simulink model "UIO_SFControl"  (R2019b)
settings: Solver=VariableStepAuto  StartTime=0.0  StopTime=1500.0  RelTol=1e-3
values from neighbouring files (symbols this model uses):
  A5 = [1 -49.59 -0.4121 4.877 0.1209; 0 0.9835 0.01639 0 0; 0 0 0.9835 0 0 ... (first row only)    [AugmentedRev1.m]    (also in DiscreteSystem.m)
  B5 = [0.85 -0.002296 0.002032; 0 0.0001374 0; 0 0.01653 0; 0 0 0.001209 ... (first row only)    [AugmentedRev1.m]    (also in DiscreteSystem.m)
  C = [1 0 0 0 0]    [AugmentedRev1.m]
  C5 = [1 0 0 0 0; 0 1 0 0 0; 0 0 1 0 0; 0 0 0 1 0; 0 0 0 0 1]    [AugmentedRev1.m]    (also in DiscreteSystem.m)
  C5_c = [1 0 0 0 0; 0 1 0 0 0; 0 0 1 0 0; 0 0 0 1 0; 0 0 0 0 1]    [AugmentedRev1.m]    (also in DiscreteSystem.m)
  D5 = [0 0 0; 0 0 0; 0 0 0; 0 0 0; 0 0 0]    [AugmentedRev1.m]    (also in DiscreteSystem.m)
  F5 = k*[1/th2 -th3 -th3 2 2]    [AugmentedRev1.m]    (also in DiscreteSystem.m)
  L = [0.0048; 0; 0; 0; 0]    [AugmentedRev1.m]
  th1 = 0.85    [AugmentedRev1.m]    (also in DiscreteSystem.m)
  th2 = 50    [AugmentedRev1.m]    (also in DiscreteSystem.m)
  th3 = 60    [AugmentedRev1.m]    (also in DiscreteSystem.m)
undefined symbols (not defined in the file or in its folder): Bu, Bu1
libraries: dspsrcs4 x2
settings Model: Creator=akshita_jain  LastModifiedBy=akshita_jain

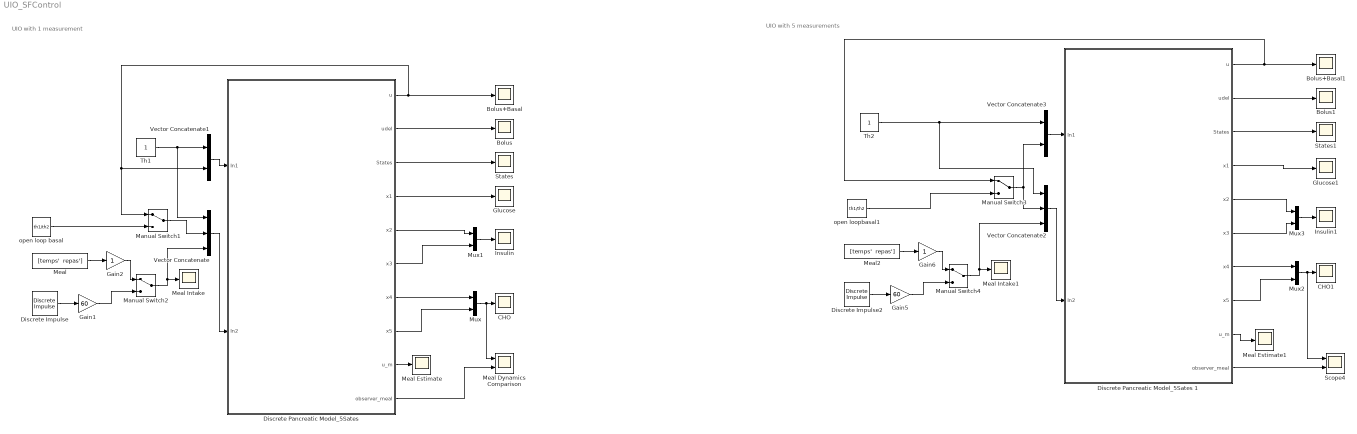
== system UIO_SFControl ==
  note: UIO with 5 measurements
  note: UIO with 1 measurement
  Bolus : Scope
  Bolus+Basal : Scope
  Bolus+Basal1 : Scope
  Bolus1 : Scope
  CHO : Scope
  CHO1 : Scope
  Discrete Impulse : dspsrcs4/Discrete  Impulse  Delay=110  SampleTime=1  FrameSample=1  OutputFrames=off  dataType=double  isSigned=on  wordLen=16  udDataType=sfix(16)  fracBitsMode=Best precision  numFracBits=15  OutDataTypeStr=double  LastOutDataTypeStr=double
  Discrete Impulse2 : dspsrcs4/Discrete  Impulse  Delay=110  SampleTime=1  FrameSample=1  OutputFrames=off  dataType=double  isSigned=on  wordLen=16  udDataType=sfix(16)  fracBitsMode=Best precision  numFracBits=15  OutDataTypeStr=double  LastOutDataTypeStr=double
  "Discrete Pancreatic Model_5Sates " : Subsystem
  Discrete Pancreatic Model_5Sates 1 : Subsystem
  Gain1 : Gain  Gain=60
  Gain2 : Gain
  Gain5 : Gain  Gain=60
  Gain6 : Gain
  Glucose : Scope
  Glucose1 : Scope
  Insulin : Scope
  Insulin1 : Scope
  Manual Switch{1..4} (4 alike) : ManualSwitch
  Meal : FromWorkspace  VariableName="[temps'  repas']"  SampleTime=0
  Meal Dynamics Comparison : Scope  NumInputPorts=2
  Meal Estimate : Scope
  Meal Estimate1 : Scope
  Meal Intake : Scope
  Meal Intake1 : Scope
  Meal2 : FromWorkspace  VariableName="[temps'  repas']"  SampleTime=0
  Mux{,1..3} (4 alike) : Mux  Inputs=2
  Scope4 : Scope  NumInputPorts=2
  States : Scope
  States1 : Scope
  Th1 : Constant
  Th2 : Constant
  Vector Concatenate : Concatenate  NumInputs=3
  Vector Concatenate1 : Concatenate
  Vector Concatenate2 : Concatenate  NumInputs=3
  Vector Concatenate3 : Concatenate
  open loop basal : Constant  Value=th1/th2
  open loopbasal1 : Constant  Value=th1/th2
  wires:
  Manual Switch1/1 -> Vector Concatenate/2
  "Discrete Pancreatic Model_5Sates "/1(u) -> Bolus+Basal/1, Manual Switch1/1, Vector Concatenate1/2
  Th1/1 -> Vector Concatenate/1, Vector Concatenate1/1
  Mux/1 -> Meal Dynamics Comparison/1, CHO/1
  "Discrete Pancreatic Model_5Sates "/4(x1) -> Glucose/1
  Discrete Impulse/1 -> Gain1/1
  "Discrete Pancreatic Model_5Sates "/9(u_m) -> Meal Estimate/1
  "Discrete Pancreatic Model_5Sates "/6(x3) -> Mux1/2
  "Discrete Pancreatic Model_5Sates "/7(x4) -> Mux/1
  open loop basal/1 -> Manual Switch1/2
  Meal/1 -> Gain2/1
  Mux1/1 -> Insulin/1
  "Discrete Pancreatic Model_5Sates "/2(udel) -> Bolus/1
  "Discrete Pancreatic Model_5Sates "/10("observer_meal ") -> Meal Dynamics Comparison/2
  "Discrete Pancreatic Model_5Sates "/5(x2) -> Mux1/1
  "Discrete Pancreatic Model_5Sates "/8(x5) -> Mux/2
  "Discrete Pancreatic Model_5Sates "/3(States) -> States/1
  Vector Concatenate/1 -> "Discrete Pancreatic Model_5Sates "/2(In2)
  Vector Concatenate1/1 -> "Discrete Pancreatic Model_5Sates "/1(In1)
  Gain1/1 -> Manual Switch2/2
  Manual Switch2/1 -> Vector Concatenate/3, Meal Intake/1
  Gain2/1 -> Manual Switch2/1
  Mux2/1 -> Scope4/1, CHO1/1
  Discrete Pancreatic Model_5Sates 1/3(States) -> States1/1
  Discrete Pancreatic Model_5Sates 1/5(x2) -> Mux3/1
  Manual Switch3/1 -> Vector Concatenate3/2, Vector Concatenate2/2
  Th2/1 -> Vector Concatenate2/1, Vector Concatenate3/1
  open loopbasal1/1 -> Manual Switch3/2
  Discrete Pancreatic Model_5Sates 1/1(u) -> Bolus+Basal1/1, Manual Switch3/1
  Discrete Pancreatic Model_5Sates 1/2(udel) -> Bolus1/1
  Discrete Pancreatic Model_5Sates 1/7(x4) -> Mux2/1
  Mux3/1 -> Insulin1/1
  Discrete Pancreatic Model_5Sates 1/4(x1) -> Glucose1/1
  Discrete Pancreatic Model_5Sates 1/6(x3) -> Mux3/2
  Discrete Pancreatic Model_5Sates 1/10("observer_meal ") -> Scope4/2
  Discrete Pancreatic Model_5Sates 1/8(x5) -> Mux2/2
  Meal2/1 -> Gain6/1
  Gain6/1 -> Manual Switch4/1
  Manual Switch4/1 -> Vector Concatenate2/3, Meal Intake1/1
  Discrete Impulse2/1 -> Gain5/1
  Gain5/1 -> Manual Switch4/2
  Vector Concatenate3/1 -> Discrete Pancreatic Model_5Sates 1/1(In1)
  Vector Concatenate2/1 -> Discrete Pancreatic Model_5Sates 1/2(In2)
  Discrete Pancreatic Model_5Sates 1/9(u_m) -> Meal Estimate1/1

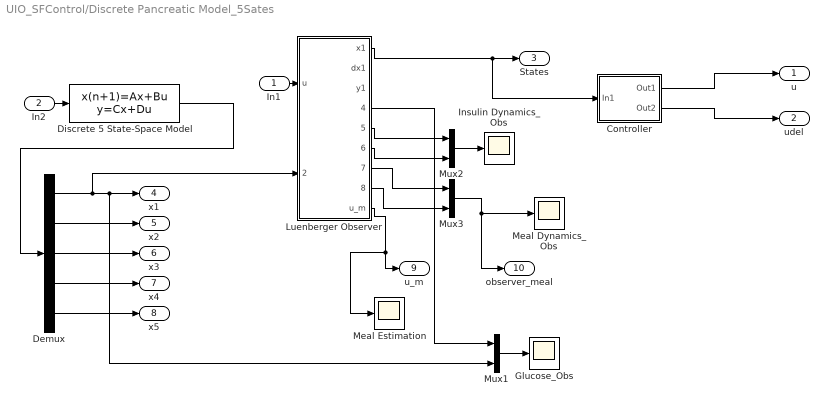
== system UIO_SFControl/Discrete Pancreatic Model_5Sates  ==
  In1 : Inport
  In2 : Inport  Port=2
  Controller : Subsystem
  Demux : Demux  Outputs=5
  Discrete 5 State-Space Model : DiscreteStateSpace  A=A5  B=B5  C=C5  D=D5  InitialCondition=[110; th1/th2; th1/th2; 0; 0]  SampleTime=-1  StateName=Glycemia
  Glucose_Obs : Scope
  Insulin Dynamics_Obs : Scope
  Luenberger Observer : Subsystem
  Meal Dynamics_Obs : Scope
  Meal Estimation : Scope
  Mux1 : Mux  Inputs=2
  Mux2 : Mux  Inputs=2
  Mux3 : Mux  Inputs=2
  u : Outport
  udel : Outport  Port=2
  States : Outport  Port=3
  x1 : Outport  Port=4
  x2 : Outport  Port=5
  x3 : Outport  Port=6
  x4 : Outport  Port=7
  x5 : Outport  Port=8
  u_m : Outport  Port=9
  "observer_meal " : Outport  Port=10
  wires:
  Discrete 5 State-Space Model/1 -> Demux/1
  Demux/5 -> x5/1
  Demux/4 -> x4/1
  Demux/3 -> x3/1
  Demux/2 -> x2/1
  Luenberger Observer/1(x1) -> Controller/1(In1), States/1
  Mux1/1 -> Glucose_Obs/1
  Luenberger Observer/4(x1_obs) -> Mux1/1
  Mux2/1 -> Insulin Dynamics_Obs/1
  Luenberger Observer/5(x2_obs) -> Mux2/1
  Luenberger Observer/6(x3_obs) -> Mux2/2
  Luenberger Observer/8(x5_obs) -> Mux3/2
  Luenberger Observer/7(x4_obs) -> Mux3/1
  Mux3/1 -> "observer_meal "/1, Meal Dynamics_Obs/1
  Demux/1 -> Luenberger Observer/2("y_plant "), Mux1/2, x1/1
  Luenberger Observer/9(u_m) -> Meal Estimation/1, u_m/1
  In2/1 -> Discrete 5 State-Space Model/1
  In1/1 -> Luenberger Observer/1(u)
  Controller/1(Out1) -> u/1
  Controller/2(Out2) -> udel/1

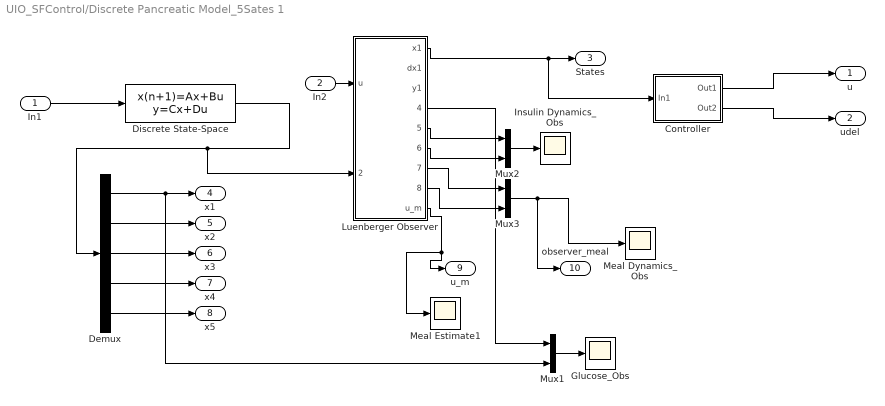
== system UIO_SFControl/Discrete Pancreatic Model_5Sates 1 ==
  In1 : Inport
  In2 : Inport  Port=2
  Controller : Subsystem
  Demux : Demux  Outputs=5
  Discrete State-Space : DiscreteStateSpace  A=A5  B=B5  C=C5  D=D5  InitialCondition=[110; th1/th2; th1/th2; 0; 0]  SampleTime=-1  StateName=Glycemia
  Glucose_Obs : Scope
  Insulin Dynamics_Obs : Scope
  Luenberger Observer : Subsystem
  Meal Dynamics_Obs : Scope
  Meal Estimate1 : Scope
  Mux1 : Mux  Inputs=2
  Mux2 : Mux  Inputs=2
  Mux3 : Mux  Inputs=2
  u : Outport
  udel : Outport  Port=2
  States : Outport  Port=3
  x1 : Outport  Port=4
  x2 : Outport  Port=5
  x3 : Outport  Port=6
  x4 : Outport  Port=7
  x5 : Outport  Port=8
  u_m : Outport  Port=9
  "observer_meal " : Outport  Port=10
  wires:
  Discrete State-Space/1 -> Luenberger Observer/2("y_plant "), Demux/1
  In1/1 -> Discrete State-Space/1
  Demux/5 -> x5/1
  Demux/4 -> x4/1
  Demux/3 -> x3/1
  Demux/2 -> x2/1
  Luenberger Observer/1(x1) -> Controller/1(In1), States/1
  Mux1/1 -> Glucose_Obs/1
  Luenberger Observer/4(x1_obs) -> Mux1/1
  Mux2/1 -> Insulin Dynamics_Obs/1
  Luenberger Observer/5(x2_obs) -> Mux2/1
  Luenberger Observer/6(x3_obs) -> Mux2/2
  Luenberger Observer/8(x5_obs) -> Mux3/2
  Luenberger Observer/7(x4_obs) -> Mux3/1
  Mux3/1 -> "observer_meal "/1, Meal Dynamics_Obs/1
  Demux/1 -> Mux1/2, x1/1
  Luenberger Observer/9(u_m) -> Meal Estimate1/1, u_m/1
  In2/1 -> Luenberger Observer/1(u)
  Controller/1(Out1) -> u/1
  Controller/2(Out2) -> udel/1

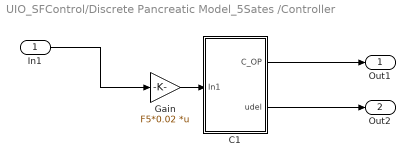
== system UIO_SFControl/Discrete Pancreatic Model_5Sates /Controller ==
  In1 : Inport
  "C1 " : Subsystem
  Gain : Gain  Gain=F5*0.02  Multiplication=Matrix(K*u)
  Out1 : Outport
  Out2 : Outport  Port=2
  wires:
  In1/1 -> Gain/1
  "C1 "/2(udel) -> Out2/1
  "C1 "/1(C_OP) -> Out1/1
  Gain/1 -> "C1 "/1(In1)

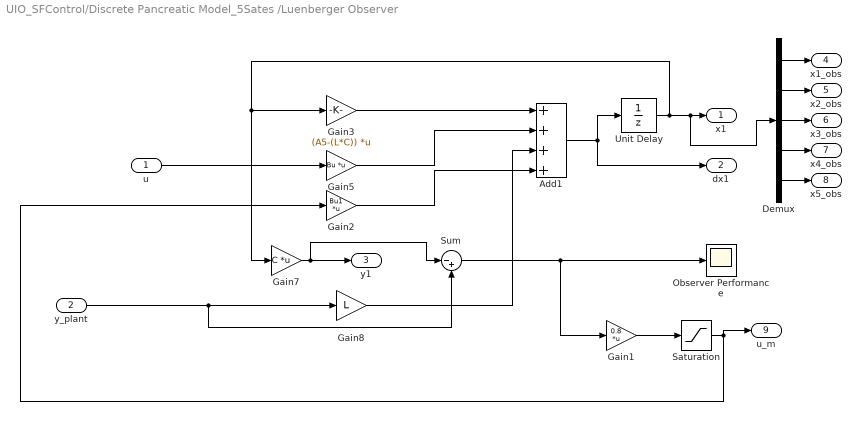
== system UIO_SFControl/Discrete Pancreatic Model_5Sates /Luenberger Observer ==
  u : Inport
  "y_plant " : Inport  Port=2
  Add1 : Sum  Inputs=4
  Demux : Demux  Outputs=5
  Gain1 : Gain  Gain=0.8  Multiplication=Matrix(K*u)
  Gain2 : Gain  Gain=Bu1  Multiplication=Matrix(K*u)
  Gain3 : Gain  Gain=(A5-(L*C))  Multiplication=Matrix(K*u)
  Gain5 : Gain  Gain=Bu  Multiplication=Matrix(K*u)
  Gain7 : Gain  Gain=C  Multiplication=Matrix(K*u)
  Gain8 : Gain  Gain=L
  Observer Performance : Scope
  Saturation : Saturate  UpperLimit=30  LowerLimit=0
  Sum : Sum  Inputs=|-+
  Unit Delay : UnitDelay  InitialCondition=[110; th1/th2; th1/th2; 0; 0]  SampleTime=-1  HasFrameUpgradeWarning=on
  x1 : Outport
  dx1 : Outport  Port=2
  y1 : Outport  Port=3
  x1_obs : Outport  Port=4
  x2_obs : Outport  Port=5
  x3_obs : Outport  Port=6
  x4_obs : Outport  Port=7
  x5_obs : Outport  Port=8
  u_m : Outport  Port=9
  wires:
  u/1 -> Gain5/1
  Sum/1 -> Gain1/1, Observer Performance/1
  Add1/1 -> Unit Delay/1, dx1/1
  Unit Delay/1 -> Demux/1, x1/1, Gain3/1, Gain7/1
  Gain3/1 -> Add1/1
  Gain8/1 -> Add1/3
  Gain7/1 -> y1/1, Sum/1
  Demux/4 -> x4_obs/1
  Demux/2 -> x2_obs/1
  Demux/3 -> x3_obs/1
  Demux/5 -> x5_obs/1
  Demux/1 -> x1_obs/1
  "y_plant "/1 -> Sum/2, Gain8/1
  Gain5/1 -> Add1/2
  Gain2/1 -> Add1/4
  Gain1/1 -> Saturation/1
  Saturation/1 -> Gain2/1, u_m/1

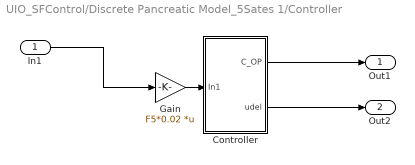
== system UIO_SFControl/Discrete Pancreatic Model_5Sates 1/Controller ==
  In1 : Inport
  "Controller " : Subsystem
  Gain : Gain  Gain=F5*0.02  Multiplication=Matrix(K*u)
  Out1 : Outport
  Out2 : Outport  Port=2
  wires:
  "Controller "/2(udel) -> Out2/1
  In1/1 -> Gain/1
  "Controller "/1(C_OP) -> Out1/1
  Gain/1 -> "Controller "/1(In1)

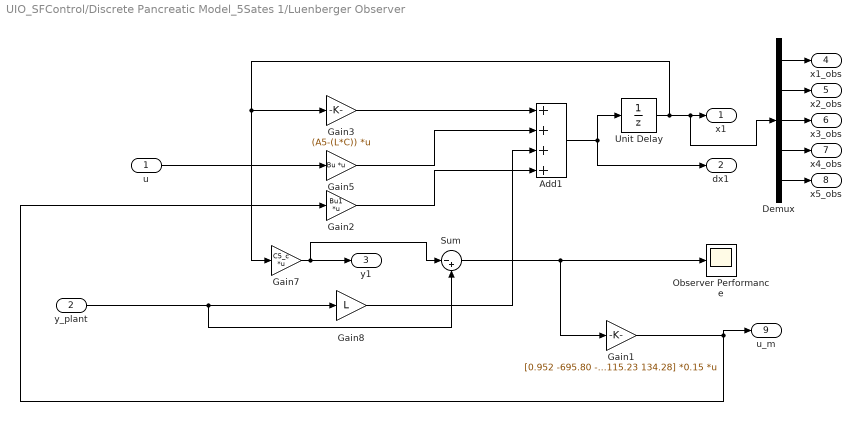
== system UIO_SFControl/Discrete Pancreatic Model_5Sates 1/Luenberger Observer ==
  u : Inport
  "y_plant " : Inport  Port=2
  Add1 : Sum  Inputs=4
  Demux : Demux  Outputs=5
  Gain1 : Gain  Gain=[0.952 -695.80 -710.02 115.23 134.28] *0.15  Multiplication=Matrix(K*u)
  Gain2 : Gain  Gain=Bu1  Multiplication=Matrix(K*u)
  Gain3 : Gain  Gain=(A5-(L*C))  Multiplication=Matrix(K*u)
  Gain5 : Gain  Gain=Bu  Multiplication=Matrix(K*u)
  Gain7 : Gain  Gain=C5_c  Multiplication=Matrix(K*u)
  Gain8 : Gain  Gain=L
  Observer Performance : Scope
  Sum : Sum  Inputs=|-+
  Unit Delay : UnitDelay  InitialCondition=[110; th1/th2; th1/th2; 0; 0]  SampleTime=-1  HasFrameUpgradeWarning=on
  x1 : Outport
  dx1 : Outport  Port=2
  y1 : Outport  Port=3
  x1_obs : Outport  Port=4
  x2_obs : Outport  Port=5
  x3_obs : Outport  Port=6
  x4_obs : Outport  Port=7
  x5_obs : Outport  Port=8
  u_m : Outport  Port=9
  wires:
  u/1 -> Gain5/1
  Sum/1 -> Gain1/1, Observer Performance/1
  Add1/1 -> Unit Delay/1, dx1/1
  Unit Delay/1 -> Demux/1, x1/1, Gain3/1, Gain7/1
  Gain3/1 -> Add1/1
  Gain8/1 -> Add1/3
  Gain7/1 -> y1/1, Sum/1
  Demux/4 -> x4_obs/1
  Demux/2 -> x2_obs/1
  Demux/3 -> x3_obs/1
  Demux/5 -> x5_obs/1
  Demux/1 -> x1_obs/1
  "y_plant "/1 -> Sum/2, Gain8/1
  Gain5/1 -> Add1/2
  Gain2/1 -> Add1/4
  Gain1/1 -> Gain2/1, u_m/1

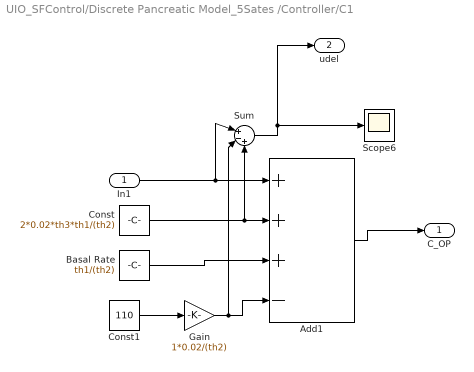
== system UIO_SFControl/Discrete Pancreatic Model_5Sates /Controller/C1  ==
  In1 : Inport
  Add1 : Sum  Inputs=+++-
  Basal Rate : Constant  Value=th1/(th2)  VectorParams1D=off
  Const : Constant  Value=2*0.02*th3*th1/(th2)  VectorParams1D=off
  Const1 : Constant  Value=110  VectorParams1D=off
  Gain : Gain  Gain=1*0.02/(th2)
  Scope6 : Scope
  Sum : Sum  Inputs=|+-+
  C_OP : Outport
  udel : Outport  Port=2
  wires:
  Const/1 -> Sum/3, Add1/2
  Basal Rate/1 -> Add1/3
  Add1/1 -> C_OP/1
  Sum/1 -> Scope6/1, udel/1
  In1/1 -> Sum/1, Add1/1
  Const1/1 -> Gain/1
  Gain/1 -> Sum/2, Add1/4

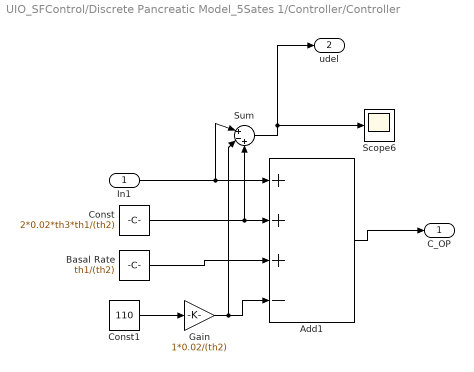
== system UIO_SFControl/Discrete Pancreatic Model_5Sates 1/Controller/Controller  ==
  In1 : Inport
  Add1 : Sum  Inputs=+++-
  Basal Rate : Constant  Value=th1/(th2)  VectorParams1D=off
  Const : Constant  Value=2*0.02*th3*th1/(th2)  VectorParams1D=off
  Const1 : Constant  Value=110  VectorParams1D=off
  Gain : Gain  Gain=1*0.02/(th2)
  Scope6 : Scope
  Sum : Sum  Inputs=|+-+
  C_OP : Outport
  udel : Outport  Port=2
  wires:
  Const/1 -> Sum/3, Add1/2
  Basal Rate/1 -> Add1/3
  Add1/1 -> C_OP/1
  Sum/1 -> Scope6/1, udel/1
  In1/1 -> Sum/1, Add1/1
  Const1/1 -> Gain/1
  Gain/1 -> Sum/2, Add1/4
